simulink model "ComputeAlgorithm_ref"  (R2023b)
settings: Solver=FixedStepAuto  StartTime=0.0  StopTime=10.0  RelTol=1e-3  EnableMultiTasking=on
libraries: prociolib x1
settings Model: Creator=lenovo GAME  LastModifiedBy=lenovo GAME
settings SolverCC: PositivePriorityOrder=on
settings DataIOCC: SaveFormat=StructureWithTime
settings OptimizationCC: EnhancedBackFolding=on  PassReuseOutputArgsAs=Individual arguments  ZeroExternalMemoryAtStartup=off  ZeroInternalMemoryAtStartup=off  MaxStackSize=64  OptimizeBlockOrder=speed  DifferentSizesBufferReuse=on  OptimizationCustomize=off  EfficientTunableParamExpr=on
settings DebuggingCC: ParameterTunabilityLossMsg=error
settings HardwareCC: ProdBitPerPointer=32  ProdBitPerSizeT=32  ProdBitPerPtrDiffT=32  ProdLargestAtomicInteger=Long  ProdLargestAtomicFloat=Double  ProdWordSize=32  ProdLongLongMode=on  ProdHWDeviceType=ARM Compatible->ARM Cortex  HardwareBoardFeatureSet=SoCBlockset
settings ModelReferenceCC: ModelReferenceNumInstancesAllowed=Single
settings SFSimCC: MATLABDynamicMemAlloc=off
settings RTWCC: Description=Embedded Coder  SystemTargetFile=ert.tlc  HardwareBoard=ZedBoard  TLCOptions="-aInlineSetEventsForThisBaseRateFcn=TLC_FALSE -aSuppressMultiTaskScheduler=TLC_FALSE  -aRateBasedStepFcn=0"  TemplateMakefile=ert_default_tmf  Toolchain=Linaro AArch32 Linux v6.3.1
settings CodeAppCC: ForceParamTrailComments=on  IgnoreCustomStorageClasses=off  OperatorAnnotations=on  SimulinkDataObjDesc=on  SFDataObjDesc=on  InsertBlockDesc=on

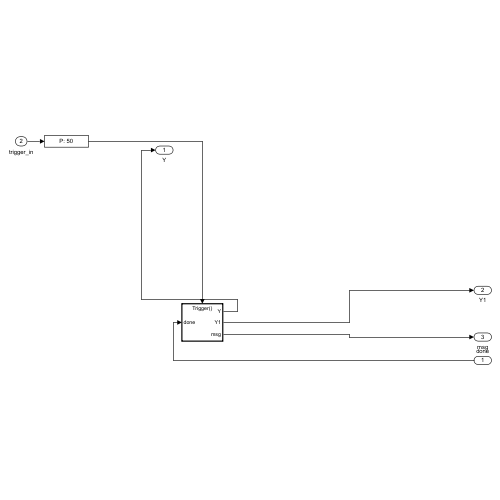
[thumbnail: Simulink's stored preview of the top-level diagram]
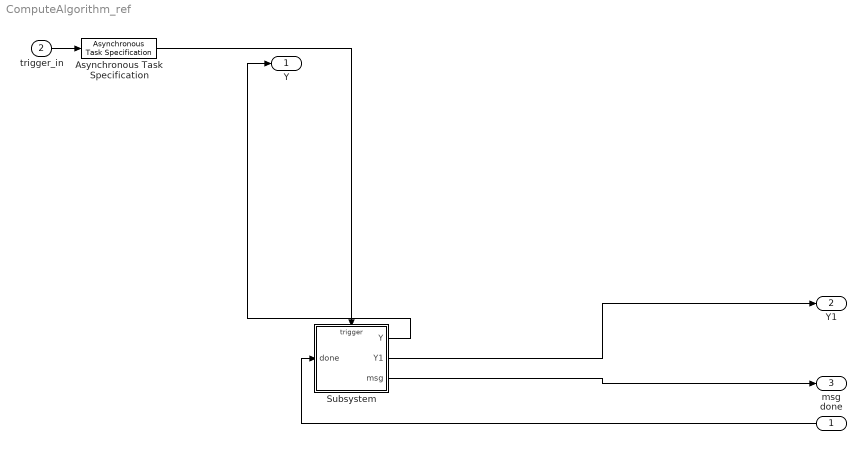
== system ComputeAlgorithm_ref ==
  done : Inport
  trigger_in : Inport  Port=2  OutputFunctionCall=on
  Asynchronous Task Specification : AsynchronousTaskSpecification  TaskPriority=50
  Subsystem : Subsystem
  Y : Outport
  Y1 : Outport  Port=2
  msg : Outport  Port=3
  wires:
  done/1 -> Subsystem/1(done)
  Subsystem/1(Y) -> Y/1
  Subsystem/2(Y1) -> Y1/1
  Subsystem/3(msg) -> msg/1
  trigger_in/1 -> Asynchronous Task Specification/1
  Asynchronous Task Specification/1 -> Subsystem/Trigger

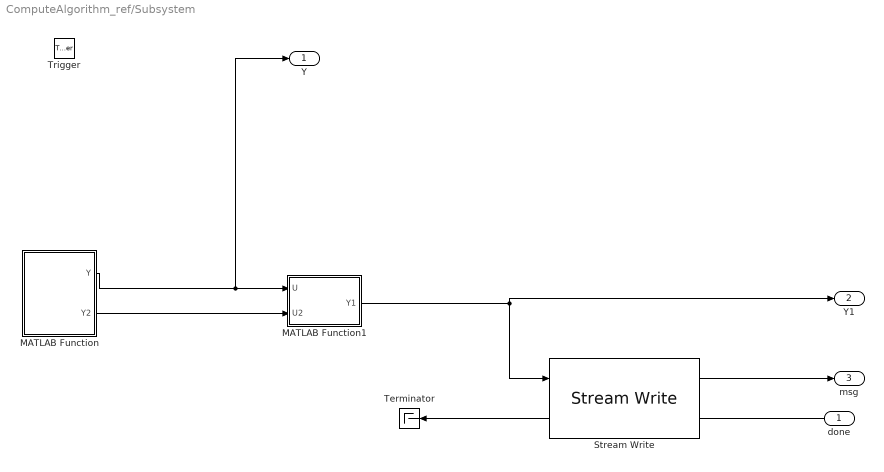
== system ComputeAlgorithm_ref/Subsystem ==
  done : Inport
  Trigger : TriggerPort  TriggerType=function-call  VariantControl=(inherit)  PortDimensions=1
  MATLAB Function : MATLAB Function  TreatAsAtomicUnit=on
  MATLAB Function1 : MATLAB Function  TreatAsAtomicUnit=on
  Stream Write : prociolib/Stream Write  DeviceName=ip:mm2s  NumberOfBuffers=8  EnableEvent=on
  Terminator : Terminator
  Y : Outport
  Y1 : Outport  Port=2
  msg : Outport  Port=3
  wires:
  MATLAB Function1/1(Y1) -> Y1/1, Stream Write/1
  Stream Write/2 -> Terminator/1
  MATLAB Function/2(Y2) -> MATLAB Function1/2(U2)
  MATLAB Function/1(Y) -> Y/1, MATLAB Function1/1(U)
  Stream Write/1 -> msg/1
  done/1 -> Stream Write/2

== matlab function ComputeAlgorithm_ref/Subsystem/MATLAB Function ==
  data: Y output; Y2 output
function [Y,Y2] = fcn()
    A = [1 2 3; 4 5 6; 7 8 9];
    B = [9 8 7; 6 5 4; 3 2 1];
    Y = A * B;
    
    C = [1 2 3 4; 5 6 7 8; 9 10 11 12; 13 14 15 16];          % o due 4x4 a piacere moltiplicate tra loro
    D = eye(4);
    Y2 = C*D;  

end

== matlab function ComputeAlgorithm_ref/Subsystem/MATLAB Function1 ==
  data: U input; Y1 output; U2 input
function Y1 = fcn(U, U2)
Y1 = [typecast(U(:),'uint64'); typecast(U2(:),'uint64')];   % 9+16 = 25 elementi
end
